simulink model "HenonHeiles"  (R2014b)
settings: Solver=ode45  StartTime=0.0  StopTime=10.0  RelTol=1e-3
values from neighbouring files (symbols this model uses):
  l = 1    [Run_HenonHeiles.m]
undefined symbols (not defined in the file or in its folder): param
settings Model: Creator=Arek  LastModifiedBy=Arek

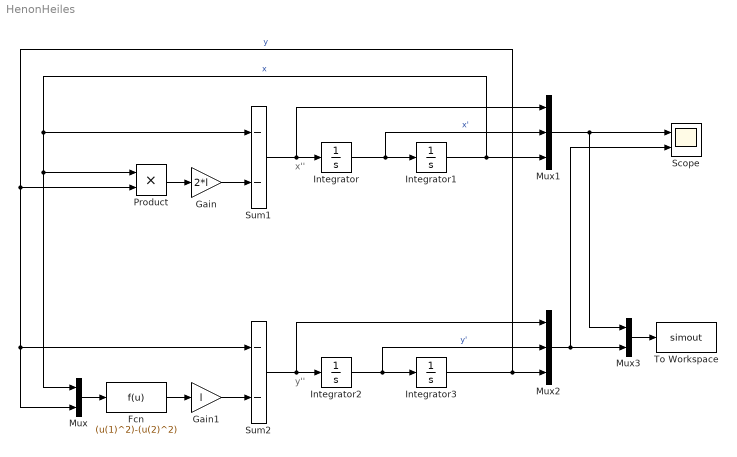
== system HenonHeiles ==
  note: x''
  note: y''
  Fcn : Fcn  Expr=(u(1)^2)-(u(2)^2)
  Gain : Gain  Gain=2*l
  Gain1 : Gain  Gain=l
  Integrator : Integrator  InitialCondition=param.ic(2)
  Integrator1 : Integrator  InitialCondition=param.ic(1)
  Integrator2 : Integrator  InitialCondition=param.ic(4)
  Integrator3 : Integrator  InitialCondition=param.ic(3)
  Mux : Mux  Inputs=2
  Mux1 : Mux  Inputs=3
  Mux2 : Mux  Inputs=3
  Mux3 : Mux  Inputs=2
  Product : Product
  Scope : Scope  NumInputPorts=2
      settings: YMin=-5~-5  YMax=5~5
  Sum1 : Sum  Inputs=--
  Sum2 : Sum  Inputs=--
  To Workspace : ToWorkspace  VariableName=simout  SaveFormat=Timeseries  SampleTime=-1
  wires:
  Integrator/1 -> Mux1/2, Integrator1/1  "x'"
  Integrator1/1 -> Mux1/3, Sum1/1, Product/1, Mux/1  "x"
  Sum1/1 -> Mux1/1, Integrator/1
  Gain/1 -> Sum1/2
  Product/1 -> Gain/1
  Integrator2/1 -> Mux2/2, Integrator3/1  "y'"
  Integrator3/1 -> Mux2/3, Product/2, Sum2/1, Mux/2  "y"
  Sum2/1 -> Mux2/1, Integrator2/1
  Gain1/1 -> Sum2/2
  Fcn/1 -> Gain1/1
  Mux/1 -> Fcn/1
  Mux2/1 -> Scope/2, Mux3/2
  Mux1/1 -> Scope/1, Mux3/1
  Mux3/1 -> To Workspace/1
